simulink model "week3prob1"  (R2020a)
settings: Solver=VariableStepAuto  StartTime=0.0  StopTime=10.0  RelTol=1e-3
settings Model: Creator=akhil singh  LastModifiedBy=akhil singh

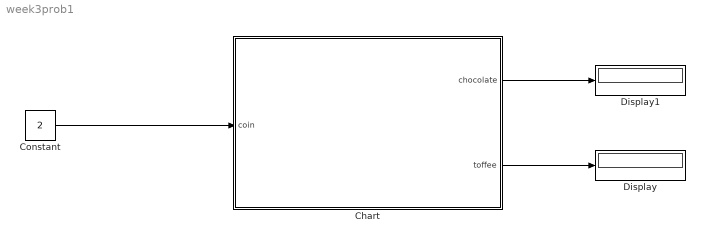
== system week3prob1 ==
  Chart : Stateflow chart  TreatAsAtomicUnit=on
  Constant : Constant  Value=2
  Display : Display
  Display1 : Display
  wires:
  Constant/1 -> Chart/1(coin)
  Chart/1(chocolate) -> Display1/1
  Chart/2(toffee) -> Display/1

== stateflow chart week3prob1/Chart ==
  state stat_1
  state nickel
  state dime
  (default) -> stat_1
  stat_1 -> nickel [order 1] : [coin==1]{toffee=0;chocolate =1;}
  nickel -> stat_1 [order 2] : [coin==2]{toffee=1}
  dime -> stat_1 [order 1] : [coin==1]{toffee=1;chocolate = 1;}
  stat_1 -> dime [order 2] : [coin==2]{toffee=0}
  nickel -> dime [order 1] : [coin==1]{toffee=0;chocolate=1;}
  dime -> nickel [order 2] : [coin==2]{toffee=1}
  data: coin input; chocolate output; toffee output
